simulink subsystem "Kalman_Filter"  (R2021a)
settings: Solver=VariableStepAuto  StartTime=0.0  StopTime=10.0  RelTol=1e-3
values from neighbouring files (symbols this model uses):
  Af = 1.6    [kf_dict.sldd]
  Cd = 0.3    [kf_dict.sldd]
  kf_A = 1.0 0.0 0.0 0.0 0.0 0.0 0.0 0.0 0.0 1.0 0.0 0.0 0.0 0.0 0.0 0.0 0.0 0.0 1.0 0.0 0.0 0.0 0.0 0.0 0.0 0.0 0.0 1.0 0.0 0.0 0.0 0.0 -0.000295833333333333 0.0 0.0 0.0 1.0 0.0 0.0 0.0 0.0 -0.000295833333333333 0.0 0.0 0.0 1.0 0.0 0.0 0.0 0.0 -0.000289029106452269 0.0 0.0 0.0 1.0 0.0 0.0 0.0 0.0 -0.000289029106452269 0.0 0.0 0.0 1.0    [kf_dict.sldd]
  kf_B = 0.001 0.0 0.0 0.0 0.0 0.0 0.0 0.0 0.0 0.001 0.0 0.0 0.0 0.0 0.0 0.0 0.0 0.0 0.001 0.0 0.0 0.0 0.0 0.0 0.0 0.0 0.0 0.001 0.0 0.0 0.0 0.0    [kf_dict.sldd]
  kf_C = 1.0 0.0 0.0 0.0 0.0 1.0 0.0 0.0 0.0 0.0 1.0 0.0 0.0 0.0 0.0 1.0 0.0 0.0 0.0 0.0 0.0 0.0 0.0 0.0 0.0 0.0 0.0 0.0 0.0 0.0 0.0 0.0    [kf_dict.sldd]
  kf_D = 0.0 0.0 0.0 0.0 0.0 0.0 0.0 0.0 0.0 0.0 0.0 0.0 0.0 0.0 0.0 0.0    [kf_dict.sldd]
  kf_L = 1.25529346077614 2.00276564441579E-17 7.41393210777867E-17 -7.67661836159404E-18 -862.96381107429 -3.75164864651043E-14 5.12295900694553E-13 -1.56315675833844E-13 8.04116153625104E-17 1.25529346077614 -1.55285428203097E-17 -2.40483552218547E-16 1.34485100686412E-15 -862.963811074287 9.38698109467505E-14 1.11031727256951E-12 6.00475947507474E-17 -1.21459165718105E-17 1.25026270665115 -1.18896732175    [kf_dict.sldd]
  kf_Psi = -0.28902910645227 0.0 0.0 0.0 0.0 0.0 0.0 0.0 0.0 -0.28902910645227 0.0 0.0 0.0 0.0 0.0 0.0 0.0 0.0 -0.28902910645227 0.0 0.0 0.0 0.0 0.0 0.0 0.0 0.0 -0.28902910645227 0.0 0.0 0.0 0.0 0.0 0.0 0.0 0.0 2.0 0.0 0.0 0.0 0.0 0.0 0.0 0.0 0.0 2.0 0.0 0.0 0.0 0.0 0.0 0.0 0.0 0.0 2.0 0.0 0.0 0.0 0.0 0.0 0.0 0.0 0.0 2.0    [kf_dict.sldd]
  rho_air = 1.206    [kf_dict.sldd]
undefined symbols (not defined in the file or in its folder): g, h, l, lf, lr, M, re
settings Model: Creator=Henrique Mesquita  LastModifiedBy=Henrique Mesquita

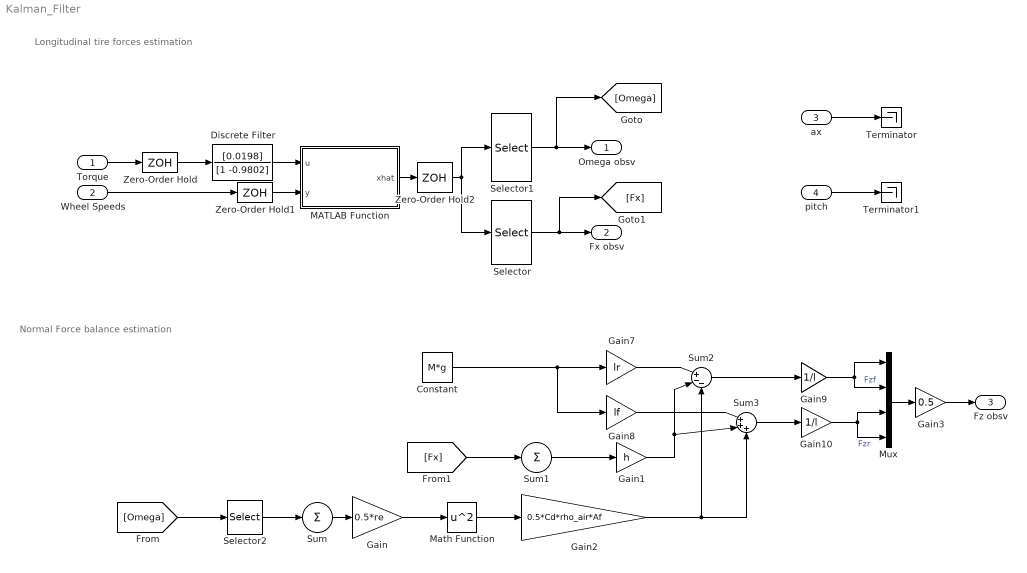
== system Kalman_Filter ==
  note: Longitudinal tire forces estimation
  note: Normal Force balance estimation
  Torque : Inport  PortDimensions=4
  Wheel Speeds : Inport  Port=2  PortDimensions=4
  ax : Inport  Port=3  PortDimensions=1
  pitch : Inport  Port=4  PortDimensions=1
  Constant : Constant  Value=M*g
  Discrete Filter : DiscreteFilter  Numerator=[0.0198]  Denominator=[1 -0.9802]  SampleTime=0.001
  Gain : Gain  Gain=0.5*re
  Gain1 : Gain  Gain=h
  Gain10 : Gain  Gain=1/l
  Gain2 : Gain  Gain=0.5*Cd*rho_air*Af
  Gain3 : Gain  Gain=0.5
  Gain7 : Gain  Gain=lr
  Gain8 : Gain  Gain=lf
  Gain9 : Gain  Gain=1/l
  MATLAB Function : MATLAB Function  TreatAsAtomicUnit=on
  Math Function : Math  Operator=square  SaturateOnIntegerOverflow=on
  Mux : Mux
  Selector : Selector  InputPortWidth=8  IndexOptions=Index vector (dialog)  Indices=[5 6 7 8]  OutputSizes=1
  Selector1 : Selector  InputPortWidth=8  IndexOptions=Index vector (dialog)  Indices=[1 2 3 4]  OutputSizes=1
  Selector2 : Selector  InputPortWidth=4  IndexOptions=Index vector (dialog)  Indices=[1 2]  OutputSizes=1
  Sum : Sum  Inputs=+
  Sum1 : Sum  Inputs=+
  Sum2 : Sum  Inputs=|+--
  Sum3 : Sum  Inputs=|+++
  Terminator : Terminator
  Terminator1 : Terminator
  Zero-Order Hold : ZeroOrderHold  SampleTime=0.001
  Zero-Order Hold1 : ZeroOrderHold  SampleTime=0.001
  Zero-Order Hold2 : ZeroOrderHold  SampleTime=0.001
  Omega obsv : Outport
  Fx obsv : Outport  Port=2
  Fz obsv : Outport  Port=3
  wires:
  Wheel Speeds/1 -> Zero-Order Hold1/1
  Selector/1 -> Fx obsv/1, [Fx]
  Selector1/1 -> Omega obsv/1, [Omega]
  MATLAB Function/1(xhat) -> Zero-Order Hold2/1
  ax/1 -> Terminator/1
  pitch/1 -> Terminator1/1
  [Omega] -> Selector2/1
  [Fx] -> Sum1/1
  Selector2/1 -> Sum/1
  Sum1/1 -> Gain1/1
  Sum/1 -> Gain/1
  Mux/1 -> Gain3/1
  Sum3/1 -> Gain10/1
  Gain10/1 -> Mux/3, Mux/4  "Fzr"
  Sum2/1 -> Gain9/1
  Gain1/1 -> Sum2/2, Sum3/2
  Gain9/1 -> Mux/1, Mux/2  "Fzf"
  Gain8/1 -> Sum3/1
  Gain7/1 -> Sum2/1
  Constant/1 -> Gain7/1, Gain8/1
  Gain/1 -> Math Function/1
  Math Function/1 -> Gain2/1
  Gain2/1 -> Sum2/3, Sum3/3
  Gain3/1 -> Fz obsv/1
  Torque/1 -> Zero-Order Hold/1
  Zero-Order Hold1/1 -> MATLAB Function/2(y)
  Zero-Order Hold2/1 -> Selector/1, Selector1/1
  Discrete Filter/1 -> MATLAB Function/1(u)
  Zero-Order Hold/1 -> Discrete Filter/1

== matlab function Kalman_Filter/MATLAB Function ==
  data: u input size=4; y input size=4; xhat output size=8; kf_L parameter; kf_A parameter; kf_B parameter; kf_C parameter; kf_D parameter; kf_Psi parameter
function xhat  = kalmanFilter(u, y, kf_L, kf_A, kf_B, kf_C, kf_D, kf_Psi)

persistent xhat_ant;    % last state
persistent y_ant;       % last output
persistent u_ant;       % last input
persistent P;
persistent R;
persistent Q;
persistent n;           % state vector size
persistent k;           % input vector size
persistent r;           % output vector size

if(isempty(xhat_ant)||isempty(y_ant)||isempty(u_ant)||isempty(n)||isempty(k)||isempty(r)||isempty(P)||isempty(Q)||isempty(R))
    n = size(kf_A,1);
    k = size(u,1);
    r = size(y,1);
    %xhat = zeros(n,1);
    xhat_ant = zeros(n,1);
    y_ant = zeros(r,1);
    u_ant = zeros(k,1);
    
    P = zeros(n);
    R = zeros(4);
    Q = [0.01*eye(4) zeros(4);zeros(4) 10000*eye(4)];
end

%current_mea_estimator = true;
% Prediction
xbar = kf_A*xhat_ant + kf_B*u;
% Correction
xhat = xbar + kf_L*(y-kf_C*xbar-kf_D*u);

% Prediction
% xbar = kf_A*xhat_ant + kf_B*u;
% M = kf_A*P*kf_A' + Q;
% % Correction
% Lc = M*kf_C'/(kf_C*M*kf_C'+R);
% xhat = xbar + Lc*(y-kf_C*xbar);
% P = (eye(n)-Lc*kf_C)*M;

xhat_ant = xhat;
u_ant = u;
y_ant = y;
